simulink model "Raeuber_Beute"  (R2020a)
settings: Solver=VariableStepAuto  StartTime=0.0  StopTime=10.0  RelTol=1e-3
values from neighbouring files (symbols this model uses):
  ax = 0.003    [test_simulink.m]    (also in ueb_simulink_Raeuber_Beute.m)
  ay = 0.002    [test_simulink.m]    (also in ueb_simulink_Raeuber_Beute.m)
  gx = 0.05    [test_simulink.m]    (also in ueb_simulink_Raeuber_Beute.m)
  gy = 0.1    [test_simulink.m]    (also in ueb_simulink_Raeuber_Beute.m)
  x_0 = 90    [test_simulink.m]    (also in ueb_simulink_Raeuber_Beute.m)
  y_0 = 15    [test_simulink.m]    (also in ueb_simulink_Raeuber_Beute.m)
settings Model: Creator=Horst  LastModifiedBy=Horst
settings DataIOCC: ReturnWorkspaceOutputs=off
settings DebuggingCC: ArithmeticOperatorsInVariantConditions=warning
settings SFSimCC: SimUseLocalCustomCode=off  CustomCodeUndefinedFunction=UseInterfaceOnly
settings RTWCC: RTWUseLocalCustomCode=off

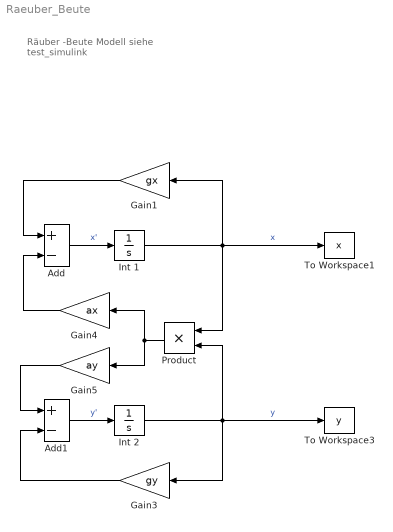
== system Raeuber_Beute ==
  note: Räuber -Beute Modell
      | siehe test_simulink
  Add : Sum  Inputs=+-
  Add1 : Sum  Inputs=+-
  Gain1 : Gain  Gain=gx
  Gain3 : Gain  Gain=gy
  Gain4 : Gain  Gain=ax
  Gain5 : Gain  Gain=ay
  Int 1 : Integrator  InitialCondition=x_0
  Int 2 : Integrator  InitialCondition=y_0
  Product : Product
  To Workspace1 : ToWorkspace  VariableName=x  SampleTime=-1
  To Workspace3 : ToWorkspace  VariableName=y  SampleTime=-1
  wires:
  Int 1/1 -> Gain1/1, To Workspace1/1, Product/1  "x"
  Add/1 -> Int 1/1  "x'"
  Gain1/1 -> Add/1
  Int 2/1 -> To Workspace3/1, Product/2, Gain3/1  "y"
  Add1/1 -> Int 2/1  "y'"
  Gain3/1 -> Add1/2
  Gain4/1 -> Add/2
  Product/1 -> Gain4/1, Gain5/1
  Gain5/1 -> Add1/1
